simulink model "mathematical_modeling2"  (R2017b)
settings: Solver=VariableStepAuto  StartTime=0.0  StopTime=40  RelTol=1e-3
values from neighbouring files (symbols this model uses):
  b1 = 1    [mathematical_modeling2_parameters.m]
  b2 = 1    [mathematical_modeling2_parameters.m]
  k1 = 5    [mathematical_modeling2_parameters.m]    (also in mathematical_modeling3_parameters.m)
  k2 = 5    [mathematical_modeling2_parameters.m]    (also in mathematical_modeling3_parameters.m)
  k3 = 5    [mathematical_modeling2_parameters.m]    (also in mathematical_modeling3_parameters.m)
  m1 = 1    [mathematical_modeling2_parameters.m]    (also in mathematical_modeling3_parameters.m)
  m2 = 3    [mathematical_modeling2_parameters.m]    (also in mathematical_modeling3_parameters.m)
  xin = 5    [mathematical_modeling2_parameters.m]
settings Model: Creator=Damla  LastModifiedBy=dagac

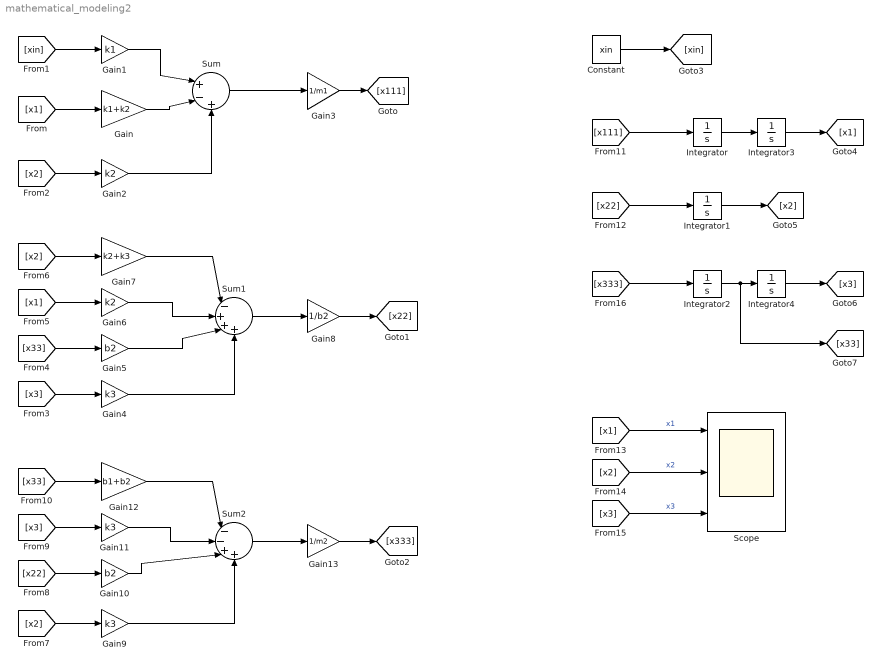
== system mathematical_modeling2 ==
  Constant : Constant  Value=xin
  Gain : Gain  Gain=k1+k2
  Gain1 : Gain  Gain=k1
  Gain10 : Gain  Gain=b2
  Gain11 : Gain  Gain=k3
  Gain12 : Gain  Gain=b1+b2
  Gain13 : Gain  Gain=1/m2
  Gain2 : Gain  Gain=k2
  Gain3 : Gain  Gain=1/m1
  Gain4 : Gain  Gain=k3
  Gain5 : Gain  Gain=b2
  Gain6 : Gain  Gain=k2
  Gain7 : Gain  Gain=k2+k3
  Gain8 : Gain  Gain=1/b2
  Gain9 : Gain  Gain=k3
  Integrator{,1..4} (5 alike) : Integrator
  Scope : Scope  NumInputPorts=3
  Sum : Sum  Inputs=|+-+
  Sum1 : Sum  Inputs=|-+++
  Sum2 : Sum  Inputs=|--++
  wires:
  [x1] -> Gain/1
  Sum/1 -> Gain3/1
  Gain3/1 -> [x111]
  [x2] -> Gain2/1
  [x3] -> Gain4/1
  [x33] -> Gain5/1
  [x1] -> Gain6/1
  [x2] -> Gain7/1
  Gain8/1 -> [x22]
  Sum1/1 -> Gain8/1
  [x3] -> Gain11/1
  [x33] -> Gain12/1
  [x2] -> Gain9/1
  Gain13/1 -> [x333]
  Sum2/1 -> Gain13/1
  [x22] -> Gain10/1
  Constant/1 -> [xin]
  [x111] -> Integrator/1
  Integrator/1 -> Integrator3/1
  Integrator3/1 -> [x1]
  Integrator2/1 -> [x33], Integrator4/1
  [x333] -> Integrator2/1
  [x22] -> Integrator1/1
  Integrator1/1 -> [x2]
  Integrator4/1 -> [x3]
  [x1] -> Scope/1  "x1"
  [x2] -> Scope/2  "x2"
  [x3] -> Scope/3  "x3"
  [xin] -> Gain1/1
  Gain1/1 -> Sum/1
  Gain/1 -> Sum/2
  Gain2/1 -> Sum/3
  Gain7/1 -> Sum1/1
  Gain4/1 -> Sum1/4
  Gain5/1 -> Sum1/3
  Gain6/1 -> Sum1/2
  Gain12/1 -> Sum2/1
  Gain11/1 -> Sum2/2
  Gain10/1 -> Sum2/3
  Gain9/1 -> Sum2/4
